simulink model "closed_loop_model"  (R2022a)
settings: Solver=VariableStepAuto  StartTime=0.0  StopTime=10.0  RelTol=1e-3
values from neighbouring files (symbols this model uses):
  G = [0.0081, 0.0872, 0.1586, -0.1202; 0.0187, 0.1826, 0.0848, -0.0224]    [workshop3.m]
settings Model: Creator=srika  LastModifiedBy=srika

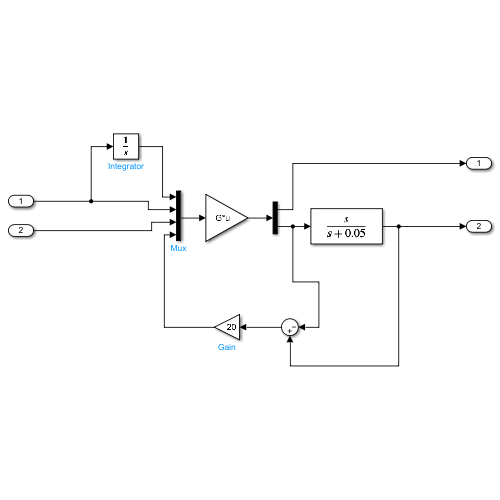
[thumbnail: Simulink's stored preview of the top-level diagram]
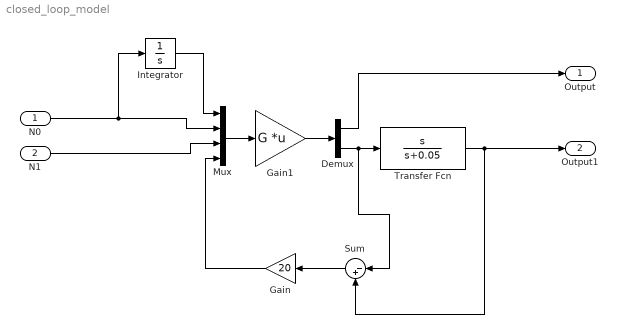
== system closed_loop_model ==
  N0 : Inport
  N1 : Inport  Port=2
  Demux : Demux  Outputs=2
  Gain : Gain  Gain=20
  Gain1 : Gain  Gain=G  Multiplication=Matrix(K*u)
  Integrator : Integrator
  Mux : Mux
  Sum : Sum  Inputs=|-+
  Transfer Fcn : TransferFcn  Numerator=[1 0]  Denominator=[1 0.05]
  Output : Outport
  Output1 : Outport  Port=2
  wires:
  Mux/1 -> Gain1/1
  Integrator/1 -> Mux/1
  N0/1 -> Integrator/1, Mux/2
  N1/1 -> Mux/3
  Transfer Fcn/1 -> Output1/1, Sum/2
  Sum/1 -> Gain/1
  Gain/1 -> Mux/4
  Gain1/1 -> Demux/1
  Demux/2 -> Sum/1, Transfer Fcn/1
  Demux/1 -> Output/1
